simulink model "mergedemo"  (Simulink 6.0)
settings: Solver=VariableStepDiscrete  SolverMode=SingleTasking  StartTime=0.0  StopTime=20  MaxStep=.1  RelTol=1e-3  AbsTol=1e-6
libraries: simulink x1
settings Model: Creator=The MathWorks Inc.  LastModifiedBy=batserve  ExtModeTrigMode=oneshot  ExtModeArmWhenConnect=off  ExtModeAutoUpdateStatusClock=off
settings DataIOCC: LimitDataPoints=off
settings OptimizationCC: BlockReduction=off
settings DebuggingCC: CheckExecutionContextPreStartOutputMsg=on  CheckExecutionContextRuntimeOutputMsg=on  SolverPrmCheckMsg=none  IntegerOverflowMsg=none
settings HardwareCC: TargetUnknown=on

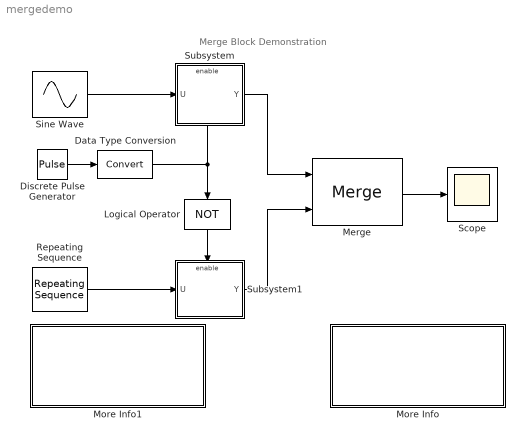
== system mergedemo ==
  note: Merge Block Demonstration
  Data Type Conversion : DataTypeConversion  OutDataTypeMode=boolean  SaturateOnIntegerOverflow=on  RndMeth=Zero
  Discrete Pulse Generator : DiscretePulseGenerator  SampleTime=5
  Logical Operator : Logic  Orientation=down  Operator=NOT  Inputs=1
  Merge : Merge
  More Info : Subsystem  PropExecContextAcrossSSBoundary=on
      settings: OpenFcn=mergedemoscript
      mask Display: disp('Double click here \nfor a step-by-step\ntutorial on this model')
  More Info1 : Subsystem  PropExecContextAcrossSSBoundary=on
      settings: OpenFcn=simcad(bdroot);
      mask Display: disp('Double click\nhere for general\nSimulink Help')
  Repeating Sequence : simulink/Sources/Repeating Sequence  rep_seq_t=[0 1]  rep_seq_y=[0 2]
  Scope : Scope
      settings: TickLabels=on  TimeRange=20  YMin=-1.5  YMax=2  DataFormat=Array
  Sine Wave : Sin  Frequency=pi  SampleTime=0
  Subsystem : Subsystem  Tag=MergeExample  TreatAsAtomicUnit=on  PropExecContextAcrossSSBoundary=on
  Subsystem1 : Subsystem  Tag=MergeExample  TreatAsAtomicUnit=on  PropExecContextAcrossSSBoundary=on
  wires:
  Sine Wave/1 -> Subsystem/1(U)
  Subsystem/1(Y) -> Merge/1
  Subsystem1/1(Y) -> Merge/2
  Logical Operator/1 -> Subsystem1/Enable
  Discrete Pulse Generator/1 -> Data Type Conversion/1
  Repeating Sequence/1 -> Subsystem1/1(U)
  Merge/1 -> Scope/1
  Data Type Conversion/1 -> Logical Operator/1, Subsystem/Enable

== system mergedemo/More Info ==
  note: Merge Block Demonstration
  note: This demonstration shows what happens when the output of two enabled
      | subsystems are merged together.  The output of the merge block is the last
      |  output written to the input ports of the block.
      |
      | While the simulation is running, the subsystem which is green is the one
      | whose signal is displayed on the scope. The coloring of the blocks is
      | controlled by an S-Function which exists in the enabled subsystems.  This
      | S-Function also artifically slows down the simulation by placing a short
      | pause in the S-Function.

== system mergedemo/More Info1 ==

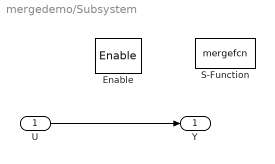
== system mergedemo/Subsystem ==
  U : Inport  Port=1  LatchInput=off
  Enable : EnablePort  StatesWhenEnabling=reset
  S-Function : S-Function  FunctionName=mergefcn
  Y : Outport
  wires:
  U/1 -> Y/1

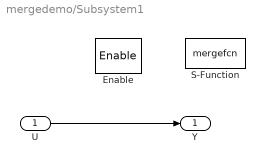
== system mergedemo/Subsystem1 ==
  U : Inport  Port=1  LatchInput=off
  Enable : EnablePort  StatesWhenEnabling=reset
  S-Function : S-Function  FunctionName=mergefcn
  Y : Outport
  wires:
  U/1 -> Y/1
